simulink model "inversor"  (R2020b)
settings: Solver=ode45  StartTime=0.0  StopTime=0.1  RelTol=1e-3  EnableMultiTasking=on
libraries: powerlib x13, powerlib_meascontrol x1
settings Model: Creator=Student  LastModifiedBy=Mateo
settings DataIOCC: LimitDataPoints=on  SaveFormat=Array  ReturnWorkspaceOutputs=off
settings OptimizationCC: LifeSpan=inf
settings DebuggingCC: UnderspecifiedInitializationDetection=Classic  MergeDetectMultiDrivingBlocksExec=none  SolverPrmCheckMsg=warning  SFUnexpectedBacktrackingDiag=warning  SFNoUnconditionalDefaultTransitionDiag=warning  SFExecutionAtInitializationDiag=none  ArithmeticOperatorsInVariantConditions=warning
settings HardwareCC: ProdBitPerPointer=32  ProdBitPerSizeT=32  ProdBitPerPtrDiffT=32  ProdLargestAtomicFloat=None  ProdIntDivRoundTo=Undefined  ProdEndianess=Unspecified  ProdWordSize=32  ProdHWDeviceType=32-bit Generic
settings ModelReferenceCC: PropagateSignalLabelsOutOfModel=off
settings SFSimCC: SimUseLocalCustomCode=off  CustomCodeUndefinedFunction=UseInterfaceOnly
settings RTWCC: RTWUseLocalCustomCode=off
settings CodeAppCC: StateflowObjectComments=on
settings GRTTargetCC: TargetLangStandard=C89/C90 (ANSI)
settings ConfigComp: CovMetricSettings=dw  CovSaveCumulativeToWorkspaceVar=on  CovSaveSingleToWorkspaceVar=on  CovExternalEMLEnable=off
settings SimscapeCC: SimscapeNormalizeSystem=off

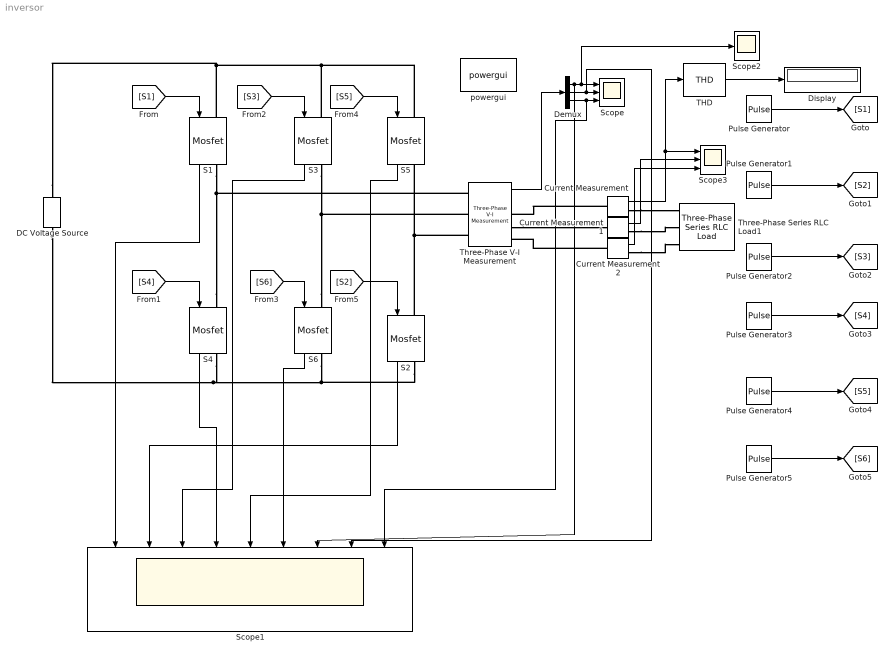
== system inversor ==
  Current Measurement : powerlib/Measurements/Current Measurement  PhasorSimulation=off  OutputType=Complex  PSBequivalent=0
  Current Measurement1 : powerlib/Measurements/Current Measurement  PhasorSimulation=off  OutputType=Complex  PSBequivalent=0
  Current Measurement2 : powerlib/Measurements/Current Measurement  PhasorSimulation=off  OutputType=Complex  PSBequivalent=0
  DC Voltage Source : powerlib/Electrical Sources/DC Voltage Source  Amplitude=220  Measurements=Voltage
  Demux : Demux  Outputs=3
  Display : Display
  Pulse Generator : DiscretePulseGenerator  PulseType=Time based  Period=1/400  PulseWidth=50
  Pulse Generator1 : DiscretePulseGenerator  PulseType=Time based  Period=1/400  PulseWidth=50  PhaseDelay=(60/400)/360
  Pulse Generator2 : DiscretePulseGenerator  PulseType=Time based  Period=1/400  PulseWidth=50  PhaseDelay=(120/400)/360
  Pulse Generator3 : DiscretePulseGenerator  PulseType=Time based  Period=1/400  PulseWidth=50  PhaseDelay=(180/400)/360
  Pulse Generator4 : DiscretePulseGenerator  PulseType=Time based  Period=1/400  PulseWidth=50  PhaseDelay=(240/400)/360
  Pulse Generator5 : DiscretePulseGenerator  PulseType=Time based  Period=1/400  PulseWidth=50  PhaseDelay=(300/400)/360
  S{1..3,5} (4 alike) : powerlib/Power Electronics/Mosfet  Ron=0.1  Lon=0  Rd=0.01  Vfd=0  IC=0  Rs=1e5  Cs=inf  Measurements=on
  "S4 " : powerlib/Power Electronics/Mosfet  Ron=0.1  Lon=0  Rd=0.01  Vfd=0  IC=0  Rs=1e5  Cs=inf  Measurements=on
  "S6 " : powerlib/Power Electronics/Mosfet  Ron=0.1  Lon=0  Rd=0.01  Vfd=0  IC=0  Rs=1e5  Cs=inf  Measurements=on
  Scope : Scope  NumInputPorts=3
  Scope1 : Scope  NumInputPorts=9
  Scope2 : Scope
  Scope3 : Scope  NumInputPorts=3
  THD : powerlib_meascontrol/Measurements/THD  Freq=60  Ts=0
  Three-Phase Series RLC Load1 : powerlib/Elements/Three-Phase Series RLC Load  LConnTagsString=A|B|C  Configuration=Y (grounded)  NominalVoltage=220  Vabc=[1e3 1e3 1e3]  Vabcp=[1e3 1e3 1e3]  NominalFrequency=400  UnbalancedPower=off  ActivePower=9680  InductivePower=1925.7748  CapacitivePower=2432.849351  Pabc=[10e3 9e3 11e3]  QLabc=[100 90 110]  QCabc=[100 90 110]  Pabcp=[10e3 9e3 11e3]  QLabcp=[100 90 110]  QCabcp=[100 90 110]  Measurements=None  LoadType=constant Z
  Three-Phase V-I Measurement : powerlib/Measurements/Three-Phase V-I Measurement  VoltageMeasurement=phase-to-phase  SetLabelV=off  LabelV=Vabc  Vpu=off  VpuLL=off  CurrentMeasurement=yes  SetLabelI=off  LabelI=Iabc  Ipu=off  Pbase=100e6  Vbase=500e3  OutputType=Complex  PhasorSimulation=off  PSBequivalent=0
  powergui : powerlib/powergui  Priority=1  SimulationMode=Discrete  SampleTime=50e-7  frequency=60  Iterations=50  frequencyindice=0  Pbase=100e6  ErrMax=1e-4  UnitsV=kV  UnitsW=MW  buscounter=0  FunctionMessages=off  echomessages=off  EnableUseOfTLC=off  CurrentSourceSwitches=off  DisableSnubberDevices=off  DisableRonSwitches=off  DisableVfSwitches=off  DisplayEquations=off  AutomaticDiscreteSolvers=off  SolverType=Tustin  Interpol=off  ExternalGateDelay=off  methode=off  Ts=0  x0status=blocks  SPID=off  SwTol=0  HookPort=off  NonlinearTolerance=1e-4  nMaxIteration=100  ContinueOnMaxIteration=off  RestoreLinks=warning  ResistiveCurrentMeasurement=off  Frange=[0:2:500]  Ylog=off  Xlog=on  ShowGrid=off  save=off  variable=ZData  structure=vab  ZoomFFT=off  StartTime=0.0  cycles=3  DisplayStyle=1  fundamental=50  FreqAxis=off  MaxFrequency=1000  frequencyindicesteady=1  RmsSteady=1  display=off
  wires:
  [S1] -> S1/1
  [S3] -> S3/1
  [S4] -> "S4 "/1
  [S6] -> "S6 "/1
  [S2] -> S2/1
  [S5] -> S5/1
  Three-Phase V-I Measurement/1 -> Demux/1
  Demux/1 -> Scope1/7, Scope2/1, Scope/1
  Demux/2 -> Scope1/8, Scope/2
  Demux/3 -> Scope1/9, Scope/3
  Pulse Generator/1 -> [S1]
  Pulse Generator1/1 -> [S2]
  Pulse Generator2/1 -> [S3]
  Pulse Generator3/1 -> [S4]
  Pulse Generator4/1 -> [S5]
  Pulse Generator5/1 -> [S6]
  S1/1 -> Scope1/1
  S2/1 -> Scope1/2
  S3/1 -> Scope1/3
  "S4 "/1 -> Scope1/4
  S5/1 -> Scope1/5
  "S6 "/1 -> Scope1/6
  Current Measurement/1 -> THD/1, Scope3/1
  Current Measurement1/1 -> Scope3/2
  Current Measurement2/1 -> Scope3/3
  THD/1 -> Display/1
  connections:
  "S6 "/RConn1 -- S2/RConn1 -- DC Voltage Source/LConn1 -- "S4 "/RConn1
  DC Voltage Source/RConn1 -- S1/LConn1 -- S3/LConn1 -- S5/LConn1
  "S4 "/LConn1 -- S1/RConn1 -- Three-Phase V-I Measurement/LConn1
  "S6 "/LConn1 -- S3/RConn1 -- Three-Phase V-I Measurement/LConn2
  Three-Phase V-I Measurement/LConn3 -- S5/RConn1 -- S2/LConn1
  Current Measurement/LConn1 -- Three-Phase V-I Measurement/RConn1
  Three-Phase V-I Measurement/RConn2 -- Current Measurement1/LConn1
  Current Measurement2/LConn1 -- Three-Phase V-I Measurement/RConn3
  Current Measurement/RConn1 -- Three-Phase Series RLC Load1/LConn1
  Current Measurement1/RConn1 -- Three-Phase Series RLC Load1/LConn2
  Current Measurement2/RConn1 -- Three-Phase Series RLC Load1/LConn3
